simulink model "adaptive_sliding_mode_control"  (R2023b)
settings: Solver=VariableStepAuto  StartTime=0.0  StopTime=tot_time  RelTol=1e-3
InitFcn:
  | addpath('TRAJECTORIES\');
  | %square_coplanar
  | circular_coplanar;
StartFcn:
  | %% Setup Video e Timer
  | videoFile = 'Adaptative_quad.avi';
  | %videoFile = 'Adaptative_circ.avi';
  | videoObj = VideoWriter(videoFile);
  | videoObj.FrameRate = 30;
  | open(videoObj);
  | assignin('base','videoObj',videoObj);
  | 
  | 
  | t = timer('ExecutionMode','fixedSpacing','Period',0.05,'StartDelay',2,...
  |           'TimerFcn',@(~,~) captureFrame(findall(0,'Type','figure','Name','UAV Animation'), videoObj));
  | start(t);
  | 
  | 
  | assignin('base','videoTimer',t);
StopFcn:
  | % Default graphics settings
  | set(0, 'DefaultTextInterpreter', 'latex')
  | set(0, 'DefaultLegendInterpreter', 'latex')
  | set(0, 'DefaultAxesTickLabelInterpreter', 'latex')
  | lw = 2;
  | 
  | plot_errors = figure('Renderer', 'painters', 'Position', [10 10 900 650]);
  | 
  | subplot(2,1,1)
  | plot(out.tout, out.err_p.signals.values(1,:), 'k-', 'Linewidth', lw ,'Color', [0.2, 0.2, 0.2]);
  | hold on
  | plot(out.tout, out.err_p.signals.values(2,:), 'k-', 'Linewidth', lw ,'Color', [1, 0, 0]);
  | hold on
  | plot(out.tout, out.err_p.signals.values(3,:), 'k-', 'Linewidth', lw ,'Color', [0, 0, 1]);
  | 
  | legend({'x-axis', 'y-axis', 'z-axis'}, ...
  |        'Location', 'southeast', ...
  |        'Orientation', 'vertical', ...
  |        'FontSize', 16);
  | 
  | 
  | %xlabel('Time [s]')
  | ylabel('$e_p$ [m]')
  | 
  | set(gca, 'FontSize',20);
  | 
  | %Grid
  | grid on
  | box on
  | 
  | 
  | %----------------------------------------------------------
  | 
  | subplot(2,1,2)
  | plot(out.tout, out.dot_err_p.signals.values(1,:), 'k-', 'Linewidth', lw ,'Color', [0.2, 0.2, 0.2]);
  | hold on
  | plot(out.tout, out.dot_err_p.signals.values(2,:), 'k-', 'Linewidth', lw ,'Color', [1, 0, 0]);
  | hold on
  | plot(out.tout, out.dot_err_p.signals.values(3,:), 'k-', 'Linewidth', lw ,'Color', [0, 0, 1]);
  | 
  | legend({'x-axis', 'y-axis', 'z-axis'}, ...
  |        'Location', 'southeast', ...
  |        'Orientation', 'vertical', ...
  |        'FontSize', 16);
  | 
  | 
  | xlabel('Time [s]')
  | ylabel('$\dot{e}_p$ [m/s]')
  | 
  | set(gca, 'FontSize',20);
  | 
  | %Grid
  | grid on
  | box on
  | 
  | %Options
  | set(gcf,'color','w');
  | set(plot_errors, 'MenuBar', 'none', 'ToolBar', 'none');
  | 
  | exportgraphics(plot_errors, 'Adaptative_lin_err_dist.pdf');
  | 
  | %--------------------------------------------------
  | plot_errors_or = figure('Renderer', 'painters', 'Position', [10 10 900 650]);
  | 
  | subplot(2,1,1)
  | plot(out.tout, out.err_eta.signals.values(1,:), 'k-', 'Linewidth', lw ,'Color', [0.2, 0.2, 0.2]);
  | hold on
  | plot(out.tout, out.err_eta.signals.values(2,:), 'k-', 'Linewidth', lw ,'Color', [1, 0, 0]);
  | hold on
  | plot(out.tout, out.err_eta.signals.values(3,:), 'k-', 'Linewidth', lw ,'Color', [0, 0, 1]);
  | 
  | legend({'x-axis', 'y-axis', 'z-axis'}, ...
  |        'Location', 'northeast', ...
  |        'Orientation', 'vertical', ...
  |        'FontSize', 16);
  | 
  | 
  | ylabel('$e_{\eta}$ [rad]')
  | 
  | set(gca, 'FontSize',20);
  | 
  | %Grid
  | grid on
  | box on
  | 
  | 
  | %----------------------------------------------------------
  | 
  | subplot(2,1,2)
  | plot(out.tout, out.dot_err_eta.signals.values(1,:), 'k-', 'Linewidth', lw ,'Color', [0.2, 0.2, 0.2]);
  | hold on
  | plot(out.tout, out.dot_err_eta.signals.values(2,:), 'k-', 'Linewidth', lw ,'Color', [1, 0, 0]);
  | hold on
  | plot(out.tout, out.dot_err_eta.signals.values(3,:), 'k-', 'Linewidth', lw ,'Color', [0, 0, 1]);
  | 
  | legend({'x-axis', 'y-axis', 'z-axis'}, ...
  |        'Location', 'northeast', ...
  |        'Orientation', 'vertical', ...
  |        'FontSize', 16);
  | 
  | xlabel('Time [s]')
  | ylabel('$\dot{e_{\eta}}$ [rad/s]')
  | 
  | set(gca, 'FontSize',20);
  | 
  | %Grid
  | grid on
  | box on
  | 
  | %Options
  | set(gcf,'color','w');
  | set(plot_errors_or, 'MenuBar', 'none', 'ToolBar', 'none');
  | 
  | exportgraphics(plot_errors_or, 'Adaptative_or_err_dist.pdf');
  | 
  | 
  | %--------------------------------------------------------------
  | 
  | 
  | plot_uT = figure('Renderer', 'painters', 'Position', [10 10 900 300]);
  | 
  | plot(out.tout, out.Uf.signals.values(:,3), 'k-', 'Linewidth', lw ,'Color', [0.2, 0.2, 0.2]);
  | 
  | ylabel('$U_f$ [N]')
  | xlabel('Time [s]')
  | 
  | 
  | set(gca, 'FontSize',20);
  | 
  | %Grid
  | grid on
  | box on
  | 
  | %Options
  | set(gcf,'color','w');
  | set(plot_pos_or, 'MenuBar', 'none', 'ToolBar', 'none');
  | 
  | exportgraphics(plot_uT, 'Adaptative_cer_Uf.pdf');
  | %---------------------------------------------------------------------
  | 
  | 
  | videoObj = evalin('base','videoObj');
  | t = evalin('base','videoTimer');
  | 
  | 
  | stop(t);
  | delete(t);
  | close(videoObj);
  | 
  | 
  | clear videoObj videoTimer
  | disp('Saved Video UAV');
undefined symbols (not defined in the file or in its folder): Ib, lin_vel_0, mass, Ts
libraries: robotcorelib x2, uavutilslib x1
settings Model: Creator=acer  LastModifiedBy=laura

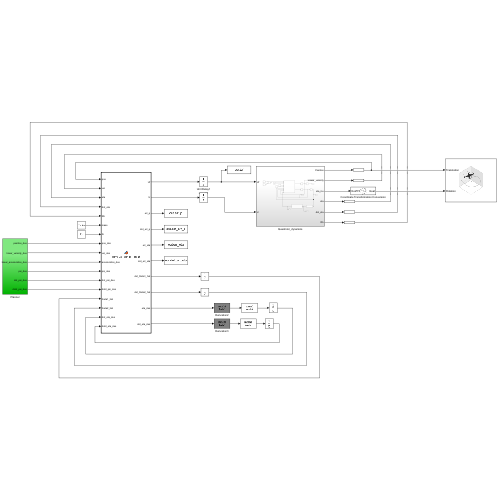
[thumbnail: Simulink's stored preview of the top-level diagram]
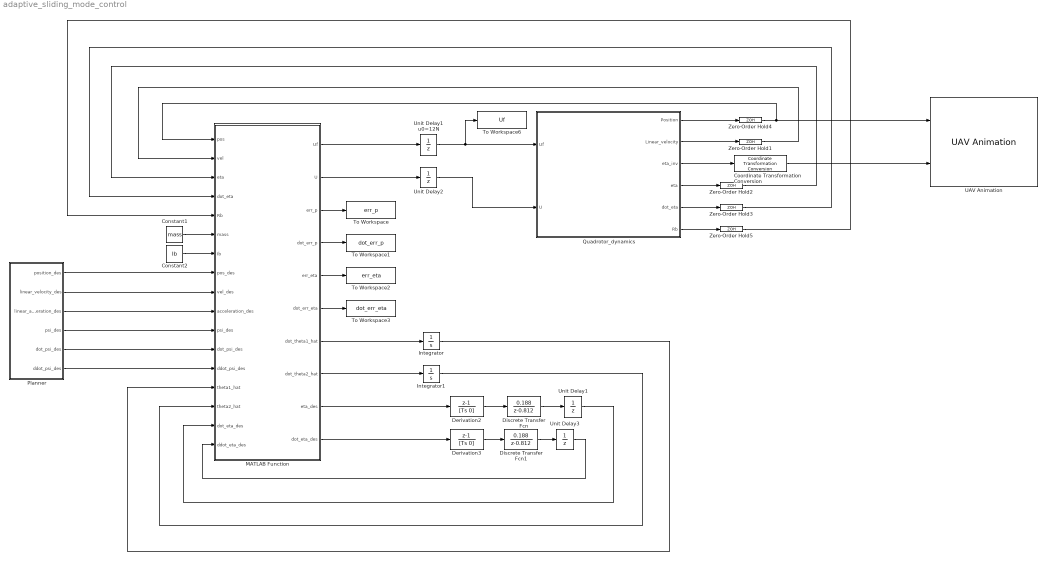
== system adaptive_sliding_mode_control ==
  Constant1 : Constant  Value=mass
  Constant2 : Constant  Value=Ib
  Coordinate Transformation Conversion : robotcorelib/Coordinate Transformation Conversion  InputRepresentation=Euler Angles  InputEulerSequence=ZYX  ShowTrVecInputPort=on  OutputRepresentation=Quaternion  OutputEulerSequence=ZYX  ShowTrVecOutputPort=on  SimulateUsing=Interpreted execution
  Derivation2 : DiscreteTransferFcn  Numerator=[1 -1]  Denominator=[Ts 0]  InitialStates=[0 0 0]'  SampleTime=Ts
  Derivation3 : DiscreteTransferFcn  Numerator=[1 -1]  Denominator=[Ts 0]  InitialStates=[0 0 0]'  SampleTime=Ts
  Discrete Transfer Fcn : DiscreteTransferFcn  Numerator=0.188  Denominator="[1  -0.812]"
  Discrete Transfer Fcn1 : DiscreteTransferFcn  Numerator=0.188  Denominator="[1  -0.812]"
  Integrator : Integrator
  Integrator1 : Integrator
  MATLAB Function : MATLAB Function  TreatAsAtomicUnit=on
  Planner : Subsystem
  Quadrotor_dynamics : Subsystem
  To Workspace : ToWorkspace  VariableName=err_p  SaveFormat=Structure With Time  SampleTime=-1
  To Workspace1 : ToWorkspace  VariableName=dot_err_p  SaveFormat=Structure With Time  SampleTime=-1
  To Workspace2 : ToWorkspace  VariableName=err_eta  SaveFormat=Structure With Time  SampleTime=-1
  To Workspace3 : ToWorkspace  VariableName=dot_err_eta  SaveFormat=Structure With Time  SampleTime=-1
  To Workspace6 : ToWorkspace  VariableName=Uf  SaveFormat=Structure With Time  SampleTime=-1
  UAV Animation : uavutilslib/UAV Animation  UAVType=Multirotor  UAVSize=1  InertialZDirection=Down  SampleTime=0.01
  Unit Delay1 : UnitDelay  InitialCondition=[0 0 0]'  SampleTime=Ts
  Unit Delay1 u0=12N : UnitDelay  InitialCondition=[0 0 12]'  SampleTime=Ts
  Unit Delay2 : UnitDelay  InitialCondition=[0 0 0]'  SampleTime=Ts
  Unit Delay3 : UnitDelay  InitialCondition=[0 0 0]'  SampleTime=Ts
  Zero-Order Hold{1..5} (5 alike) : ZeroOrderHold  SampleTime=Ts
  wires:
  Unit Delay1 u0=12N/1 -> To Workspace6/1, Quadrotor_dynamics/1(Uf)
  Zero-Order Hold4/1 -> MATLAB Function/1(pos), UAV Animation/1
  Quadrotor_dynamics/1(Position) -> Zero-Order Hold4/1
  Unit Delay2/1 -> Quadrotor_dynamics/2(U)
  Quadrotor_dynamics/2(Linear_velocity) -> Zero-Order Hold1/1
  Quadrotor_dynamics/3(eta_inv) -> Coordinate Transformation Conversion/1
  Coordinate Transformation Conversion/1 -> UAV Animation/2
  Discrete Transfer Fcn/1 -> Unit Delay1/1
  Derivation3/1 -> Discrete Transfer Fcn1/1
  Derivation2/1 -> Discrete Transfer Fcn/1
  Discrete Transfer Fcn1/1 -> Unit Delay3/1
  Quadrotor_dynamics/4(eta) -> Zero-Order Hold2/1
  Quadrotor_dynamics/5(dot_eta) -> Zero-Order Hold3/1
  MATLAB Function/7(dot_theta1_hat) -> Integrator/1
  MATLAB Function/8(dot_theta2_hat) -> Integrator1/1
  Constant1/1 -> MATLAB Function/6(mass)
  MATLAB Function/1(Uf) -> Unit Delay1 u0=12N/1
  MATLAB Function/2(U) -> Unit Delay2/1
  MATLAB Function/9(eta_des) -> Derivation2/1
  MATLAB Function/10(dot_eta_des) -> Derivation3/1
  Constant2/1 -> MATLAB Function/7(Ib)
  Planner/1(position_des) -> MATLAB Function/8(pos_des)
  Planner/2(linear_velocity_des) -> MATLAB Function/9(vel_des)
  Planner/3(linear_acceleration_des) -> MATLAB Function/10(acceleration_des)
  Planner/4(psi_des) -> MATLAB Function/11(psi_des)
  Planner/5(dot_psi_des) -> MATLAB Function/12(dot_psi_des)
  Planner/6(ddot_psi_des) -> MATLAB Function/13(ddot_psi_des)
  Unit Delay1/1 -> MATLAB Function/16("dot_eta_des ")
  Unit Delay3/1 -> MATLAB Function/17(ddot_eta_des)
  Zero-Order Hold1/1 -> MATLAB Function/2(vel)
  Zero-Order Hold2/1 -> MATLAB Function/3(eta)
  Zero-Order Hold3/1 -> MATLAB Function/4(dot_eta)
  Zero-Order Hold5/1 -> MATLAB Function/5(Rb)
  MATLAB Function/3(err_p) -> To Workspace/1
  MATLAB Function/4(dot_err_p) -> To Workspace1/1
  MATLAB Function/5(err_eta) -> To Workspace2/1
  MATLAB Function/6(dot_err_eta) -> To Workspace3/1
  Integrator1/1 -> MATLAB Function/15(theta2_hat)
  Integrator/1 -> MATLAB Function/14(theta1_hat)
  Quadrotor_dynamics/6(Rb) -> Zero-Order Hold5/1

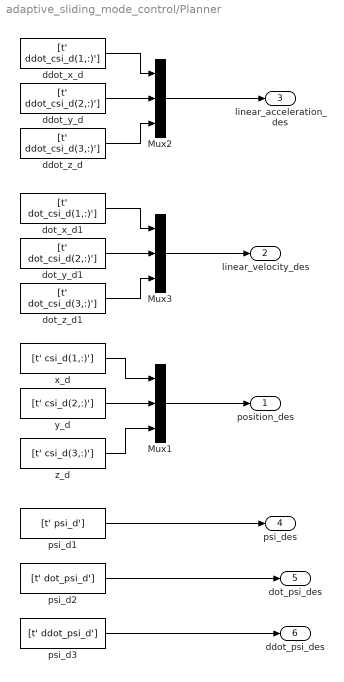
== system adaptive_sliding_mode_control/Planner ==
  Mux1 : Mux  Inputs=3
  Mux2 : Mux  Inputs=3
  Mux3 : Mux  Inputs=3
  ddot_x_d : FromWorkspace  VariableName=[t' ddot_csi_d(1,:)']  SampleTime=Ts
  ddot_y_d : FromWorkspace  VariableName=[t' ddot_csi_d(2,:)']  SampleTime=Ts
  ddot_z_d : FromWorkspace  VariableName=[t' ddot_csi_d(3,:)']  SampleTime=Ts
  dot_x_d1 : FromWorkspace  VariableName=[t' dot_csi_d(1,:)']  SampleTime=Ts
  dot_y_d1 : FromWorkspace  VariableName=[t' dot_csi_d(2,:)']  SampleTime=Ts
  dot_z_d1 : FromWorkspace  VariableName=[t' dot_csi_d(3,:)']  SampleTime=Ts
  psi_d1 : FromWorkspace  VariableName=[t' psi_d']  SampleTime=Ts
  psi_d2 : FromWorkspace  VariableName=[t' dot_psi_d']  SampleTime=Ts
  psi_d3 : FromWorkspace  VariableName=[t' ddot_psi_d']  SampleTime=Ts
  x_d : FromWorkspace  VariableName=[t' csi_d(1,:)']  SampleTime=Ts
  y_d : FromWorkspace  VariableName=[t' csi_d(2,:)']  SampleTime=Ts
  z_d : FromWorkspace  VariableName=[t' csi_d(3,:)']  SampleTime=Ts
  position_des : Outport
  linear_velocity_des : Outport  Port=2
  linear_acceleration_des : Outport  Port=3
  psi_des : Outport  Port=4
  dot_psi_des : Outport  Port=5
  ddot_psi_des : Outport  Port=6
  wires:
  y_d/1 -> Mux1/2
  z_d/1 -> Mux1/3
  x_d/1 -> Mux1/1
  ddot_y_d/1 -> Mux2/2
  ddot_z_d/1 -> Mux2/3
  ddot_x_d/1 -> Mux2/1
  Mux2/1 -> linear_acceleration_des/1
  Mux1/1 -> position_des/1
  dot_y_d1/1 -> Mux3/2
  dot_z_d1/1 -> Mux3/3
  dot_x_d1/1 -> Mux3/1
  Mux3/1 -> linear_velocity_des/1
  psi_d1/1 -> psi_des/1
  psi_d3/1 -> ddot_psi_des/1
  psi_d2/1 -> dot_psi_des/1

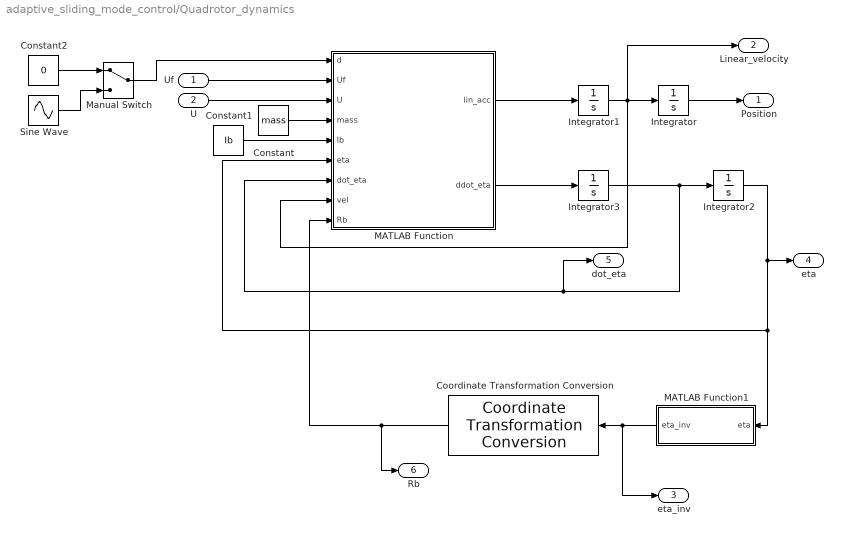
== system adaptive_sliding_mode_control/Quadrotor_dynamics ==
  Uf : Inport
  U : Inport  Port=2
  Constant : Constant  Value=mass
  Constant1 : Constant  Value=Ib
  Constant2 : Constant  Value=0
  Coordinate Transformation Conversion : robotcorelib/Coordinate Transformation Conversion  InputRepresentation=Euler Angles  InputEulerSequence=ZYX  ShowTrVecInputPort=on  OutputRepresentation=Rotation Matrix  OutputEulerSequence=ZYX  ShowTrVecOutputPort=on  SimulateUsing=Interpreted execution
  Integrator : Integrator  InitialCondition=[0 0 -1]'
  Integrator1 : Integrator  InitialCondition=lin_vel_0'
  Integrator2 : Integrator  InitialCondition=[0,0,0]'
  Integrator3 : Integrator  InitialCondition=[0 0 0]'
  MATLAB Function : MATLAB Function  TreatAsAtomicUnit=on
  MATLAB Function1 : MATLAB Function  TreatAsAtomicUnit=on
  Manual Switch : ManualSwitch
  Sine Wave : Sin  Frequency=0.2  SampleTime=0
  Position : Outport
  Linear_velocity : Outport  Port=2
  eta_inv : Outport  Port=3
  eta : Outport  Port=4
  dot_eta : Outport  Port=5
  Rb : Outport  Port=6
  wires:
  U/1 -> MATLAB Function/3(U)
  Integrator/1 -> Position/1
  MATLAB Function/1(lin_acc) -> Integrator1/1
  Uf/1 -> MATLAB Function/2(Uf)
  Integrator1/1 -> Linear_velocity/1, Integrator/1, MATLAB Function/8(vel)
  Integrator3/1 -> dot_eta/1, MATLAB Function/7(dot_eta), Integrator2/1
  MATLAB Function/2(ddot_eta) -> Integrator3/1
  Constant/1 -> MATLAB Function/4(mass)
  Constant1/1 -> MATLAB Function/5(Ib)
  Integrator2/1 -> MATLAB Function1/1(eta), MATLAB Function/6(eta), eta/1
  MATLAB Function1/1(eta_inv) -> eta_inv/1, Coordinate Transformation Conversion/1
  Coordinate Transformation Conversion/1 -> Rb/1, MATLAB Function/9(Rb)
  Constant2/1 -> Manual Switch/1
  Manual Switch/1 -> MATLAB Function/1(d)
  Sine Wave/1 -> Manual Switch/2

== matlab function adaptive_sliding_mode_control/Quadrotor_dynamics/MATLAB Function1 ==
  data: eta input; eta_inv output
function eta_inv = fcn(eta)

eta_inv = [eta(3) eta(2) eta(1)]';

== matlab function adaptive_sliding_mode_control/Quadrotor_dynamics/MATLAB Function ==
  data: d input; Uf input; lin_acc output; U input; mass input; Ib input; eta input; dot_eta input; ddot_eta output; vel input; Rb input
function [lin_acc,ddot_eta] = fcn(d,Uf,U,mass, Ib , eta, dot_eta, vel,Rb)
    
    
    L = diag([0.48 1.2 1.44]);
    lin_acc = inv(mass*Rb')*Uf -(1/mass)*L*vel - 9.81*[0 0 1]'+d*ones(3,1);
    B = [1 0 -sin(eta(2));0 cos(eta(1)) cos(eta(2))*sin(eta(1));0 -sin(eta(1)) cos(eta(1))*cos(eta(2))];

    D = [-cos(eta(2))*dot_eta(2)*dot_eta(3);
         -sin(eta(1))*dot_eta(1)*dot_eta(2)+cos(eta(1))*cos(eta(2))*dot_eta(1)*dot_eta(3)-sin(eta(1))*sin(eta(2))*dot_eta(2)*dot_eta(3);
         -cos(eta(1))*dot_eta(1)*dot_eta(2)-sin(eta(1))*cos(eta(2))*dot_eta(1)*dot_eta(3)-cos(eta(1))*sin(eta(2))*dot_eta(2)*dot_eta(3)];
    Ma = diag([1.8624 2.0735 1.4899]);

    omega = B*dot_eta;

    prod_vec1 = [omega(2)*Ib(3,3)*omega(3)-omega(3)*Ib(2,2)*omega(2);
                 omega(3)*Ib(1,1)*omega(1)-omega(1)*Ib(3,3)*omega(3);
                 omega(1)*Ib(2,2)*omega(2)-omega(2)*Ib(1,1)*omega(1)];

    cf   = 1.65776e-5;
    cm   = 2.1792e-7;
    l    = 0.45;

    A = [-cf -cf -cf -cf;0 -l*cf 0 -l*cf;l*cf 0 -l*cf 0;-cm cm -cm cm];

    T = -Uf'*Rb(:,3);
    F = pinv(A)*[T;U];

    F1 = max(0, F(1));
    F2 = max(0, F(2));
    F3 = max(0, F(3));
    F4 = max(0, F(4));

    w1 = sqrt(F1);
    w2 = sqrt(F2);
    w3 = sqrt(F3);
    w4 = sqrt(F4);

    Ir = diag([0.5*10e-4 0.5*10e-4 0.5*10e-4]);
    sum = Ir(1,1)*(-w1+w2-w3+w4);

    prod_vec2 = [omega(2)*sum;-omega(1)*sum;0];

    ddot_eta = inv(Ib*B)*U - inv(B)*D - inv(Ib)*Ma*dot_eta - prod_vec1 - prod_vec2 ;
 
end


function S = skew(v)
if(numel(v)~= 1)
S= [0 -v(3) v(2);
    v(3) 0 -v(1);
    -v(2) v(1) 0];
else
S= zeros(3);
end
end

== matlab function adaptive_sliding_mode_control/MATLAB Function ==
  data: pos input; vel input; eta input; dot_eta input; Rb input; mass input; Uf output; Ib input; pos_des input; vel_des input; acceleration_des input; psi_des input; dot_psi_des input; ddot_psi_des input; theta1_hat input; theta2_hat input; dot_eta_des input; ddot_eta_des input; U output; err_p output; dot_err_p output; err_eta output; dot_err_eta output; dot_theta1_hat output; dot_theta2_hat output; eta_des output; dot_eta_des output
function [Uf, U, err_p, dot_err_p, err_eta, dot_err_eta, dot_theta1_hat, dot_theta2_hat, eta_des, dot_eta_des] = compute_control_input(pos, vel, eta, dot_eta, Rb, mass, Ib, ...
pos_des, vel_des, acceleration_des, psi_des, dot_psi_des, ddot_psi_des, theta1_hat, theta2_hat, dot_eta_des, ddot_eta_des)
    
    %Compute linear errors
    err_p = pos_des - pos;
    dot_err_p = vel_des - vel;

    g = 9.81;
    gamma = [0 0 g]';
    L = diag([0.48 1.2 1.44]);
    B = [1 0 -sin(eta(2));0 cos(eta(1)) cos(eta(2))*sin(eta(1));0 -sin(eta(1)) cos(eta(1))*cos(eta(2))];
    
    %Gains
    lambda_L = diag([20 20 50]);
    kL = diag([20 20 50]);
    Gamma1 = 0.001;
    Gamma2 = 0.001;
    lambda_A = diag([5 5 10]);
    kA = diag([5 5 10]);
    
    %Component for the control on the angular dynamics
    SL = dot_err_p + lambda_L*err_p;
    dot_theta1_hat = Gamma1*SL'*sign(SL);
    ul = theta1_hat*sign(SL);
    Uf = (mass*Rb')*(acceleration_des + (1/mass)*L*vel + lambda_L*dot_err_p + gamma + kL*SL - ul);
    
    %Computation of desired roll and pitch checking that the argument of asin is less or equal of 1 in module
    Uf1 = Uf(1)/Uf(3);
    Uf2 = Uf(2)/Uf(3);
    z_phi = Uf1*sin(psi_des) - Uf2*cos(psi_des);
    z_phi = min(max(z_phi, -1), 1);  % protezione asin
    phi_d = asin(z_phi);
    z = (Uf1*cos(psi_des) + Uf2*sin(psi_des)) / cos(psi_des);
    z = min(max(z, -1), 1);  % per sicurezza
    theta_d = asin(z);
    
    eta_des = [phi_d theta_d psi_des]';

    % We replace the derivative values computed numerically with those provided by the trajectory planner, which are more accurate and not affected by numerical differentiation errors.
    dot_eta_des(3) = dot_psi_des;
    ddot_eta_des(3) = ddot_psi_des;
    
    %Compute angular errors
    err_eta = eta_des - eta;
    dot_err_eta = dot_eta_des - dot_eta;
    
    %Component for the control on the angular dynamics
    SA = dot_err_eta + lambda_A*err_eta;
    dot_theta2_hat = Gamma2*SA'*sign(SA);
    uA = theta2_hat*sign(SA);
    U = Ib*B*(ddot_eta_des + lambda_A*dot_err_eta + kA*SA - uA);

end
